simulink model "Eq4_CapacityCorrectionFactor"  (R2022b)
settings: Solver=FixedStepAuto  StartTime=0.0  StopTime=10.0  RelTol=1e-3
settings Model: Creator=umber  LastModifiedBy=umber
settings OptimizationCC: OptimizeBlockIOStorage=off  OptimizeDataStoreBuffers=off  BusAssignmentInplaceUpdate=off
settings DebuggingCC: SFUnexpectedBacktrackingDiag=warning  SFNoUnconditionalDefaultTransitionDiag=warning
settings ModelReferenceCC: EnableRefExpFcnMdlSchedulingChecks=on
settings RTWCC: GenCodeOnly=on  GenerateReport=on  BuildConfiguration=Debug  LaunchReport=on
settings CodeAppCC: ForceParamTrailComments=on  MATLABSourceComments=on  EnableCustomComments=on
settings GRTTargetCC: CombineSignalStateStructs=on  SupportVariableSizeSignals=on  MultiInstanceErrorCode=Warning

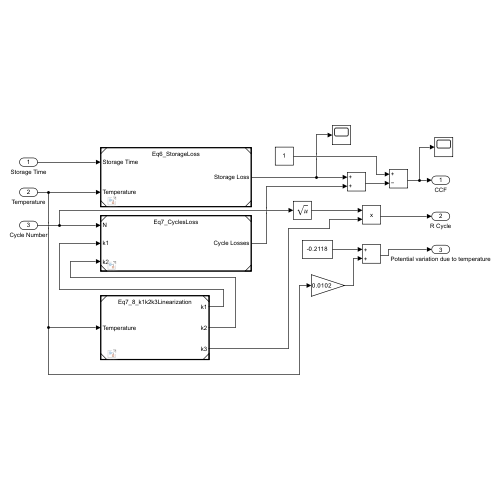
[thumbnail: Simulink's stored preview of the top-level diagram]
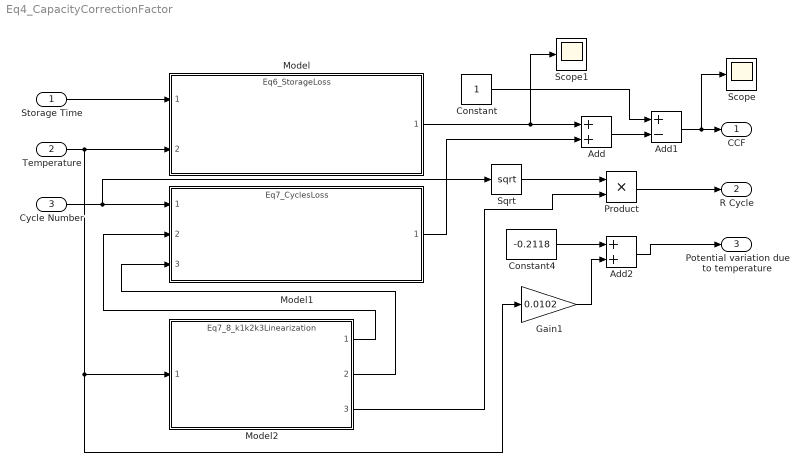
== system Eq4_CapacityCorrectionFactor ==
  Storage Time : Inport
  Temperature : Inport  Port=2
  Cycle Number : Inport  Port=3
  Add : Sum
  Add1 : Sum  Inputs=+-
  Add2 : Sum
  Constant : Constant
  Constant4 : Constant  Value=-0.2118
  Gain1 : Gain  Gain=0.0102
  Model : ModelReference  ModelNameDialog=Eq6_StorageLoss.slx  SimulationMode=Normal  ModelReferenceVersion=2.9
  Model1 : ModelReference  ModelNameDialog=Eq7_CyclesLoss.slx  SimulationMode=Normal  ModelReferenceVersion=2.4
  Model2 : ModelReference  ModelNameDialog=Eq7_8_k1k2k3Linearization.slx  SimulationMode=Normal  ModelReferenceVersion=1.6
  Product : Product
  Scope : Scope
  Scope1 : Scope
  Sqrt : Sqrt
  CCF : Outport
  R Cycle : Outport  Port=2
  Potential variation due to temperature : Outport  Port=3
  wires:
  Model/1 -> Scope1/1, Add/1
  Model1/1 -> Add/2
  Add/1 -> Add1/2
  Constant/1 -> Add1/1
  Add1/1 -> Scope/1, CCF/1
  Storage Time/1 -> Model/1
  Temperature/1 -> Model/2, Model2/1, Gain1/1
  Cycle Number/1 -> Sqrt/1, Model1/1
  Add2/1 -> Potential variation due to temperature/1
  Constant4/1 -> Add2/1
  Gain1/1 -> Add2/2
  Model2/1 -> Model1/2
  Model2/2 -> Model1/3
  Model2/3 -> Product/2
  Sqrt/1 -> Product/1
  Product/1 -> R Cycle/1
